simulink model "Simple_Model"  (R2023a)
settings: Solver=VariableStepAuto  StartTime=0.0  StopTime=60  RelTol=1e-3
settings Model: Creator=amann  LastModifiedBy=amann

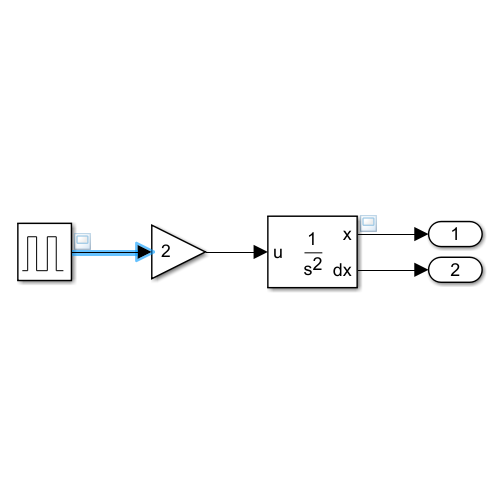
[thumbnail: Simulink's stored preview of the top-level diagram]
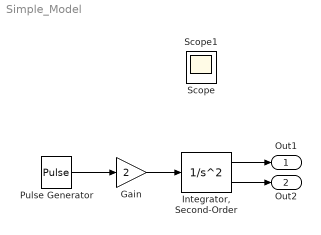
== system Simple_Model ==
  Gain : Gain  Gain=2
  "Integrator, Second-Order" : SecondOrderIntegrator
  Pulse Generator : DiscretePulseGenerator  PulseType=Time based  Period=10  PulseWidth=5
  Out1 : Outport
  Out2 : Outport  Port=2
  Scope : Scope
  Scope1 : Scope
  wires:
  Gain/1 -> "Integrator, Second-Order"/1
  Pulse Generator/1 -> Gain/1
  "Integrator, Second-Order"/1 -> Out1/1
  "Integrator, Second-Order"/2 -> Out2/1
